simulink model "Wind_Disturbances"  (R2021b)
settings: Solver=VariableStepAuto  StartTime=0.0  StopTime=10.0  RelTol=1e-3
settings Model: Creator=hpShe  LastModifiedBy=hpShe

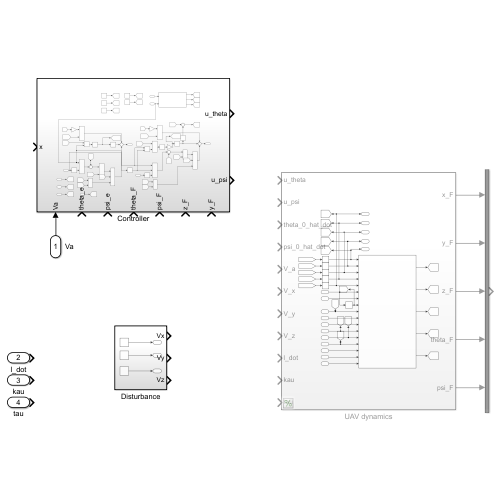
[thumbnail: Simulink's stored preview of the top-level diagram]
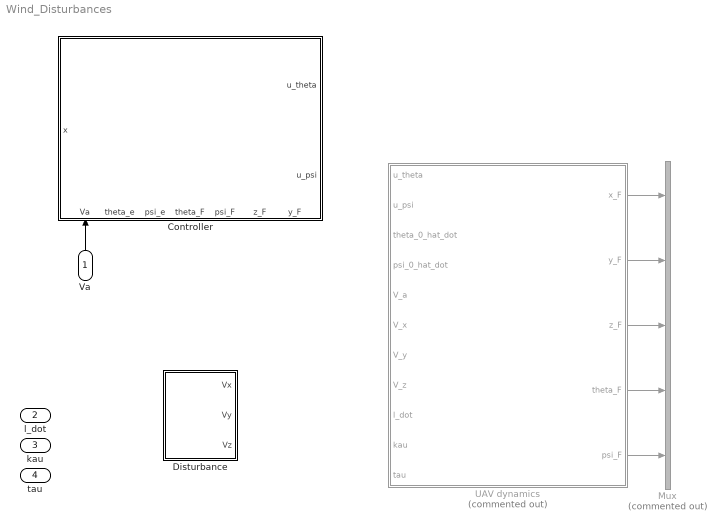
== system Wind_Disturbances ==
  Va : Inport
  l_dot : Inport  Port=2
  kau : Inport  Port=3
  tau : Inport  Port=4
  Controller : Subsystem
      settings: PortSchema="{\"entries\":[{\"content\":{\"sides\":[{\"content\":{\"connectorIds\":[\"In1\"]},\"type\":\"ConnectorPlacement.EquallySpacedRectSide\",\"uuid\":\"85cc706c-7fbb-4ce6-ac6b-8f90726b5cac\"},{\"content\":{\"connectorIds\":[\"Out1\",\"Out2\"],\"side\":\"RIGHT\"},\"type\":\"ConnectorPlacement.EquallySpacedRectSide\",\"uuid\":\"6892ba77-39c0-4603-ac59-cd93350c5557\"},{\"content\":{\"connectorIds\":[],\"side\":\"TOP\"},\"type\":\"ConnectorPlacement.EquallySpacedRectSide\",\"uuid\":\"746b4133-f075-4f92-bb9b-9c21b536ab13\"},{\"content\":{\"connectorIds\":[\"In2\",\"In3\",\"In4\",\"In5\",\"In6\",\"In7\",\"In8\"],\"side\":\"BOTTOM\"},\"type\":\"ConnectorPlacement.EquallySpacedRectSide\",\"uuid\":\"759ff651-9d48-4794-8429-93ccccddab8e\"}]},\"type\":\"ConnectorPlacement.EquallySpacedConnector\",\"uuid\":\"962f8f2c-dfce-46e4-be1a-2f59c37604ab\"}],\"packageUris\":[\"http://schema.mathworks.com/mf0/Connector/R2020b\"],\"version\":\"1.0\"}"
  Disturbance : Subsystem
  Mux : Mux  Commented=on  Inputs=5
  UAV dynamics : Subsystem  Commented=on
  wires:
  Va/1 -> Controller/2(Va)
  UAV dynamics/1(x_F) -> Mux/1
  UAV dynamics/2(y_F) -> Mux/2
  UAV dynamics/3(z_F) -> Mux/3
  UAV dynamics/4(theta_F) -> Mux/4
  UAV dynamics/5(psi_F) -> Mux/5

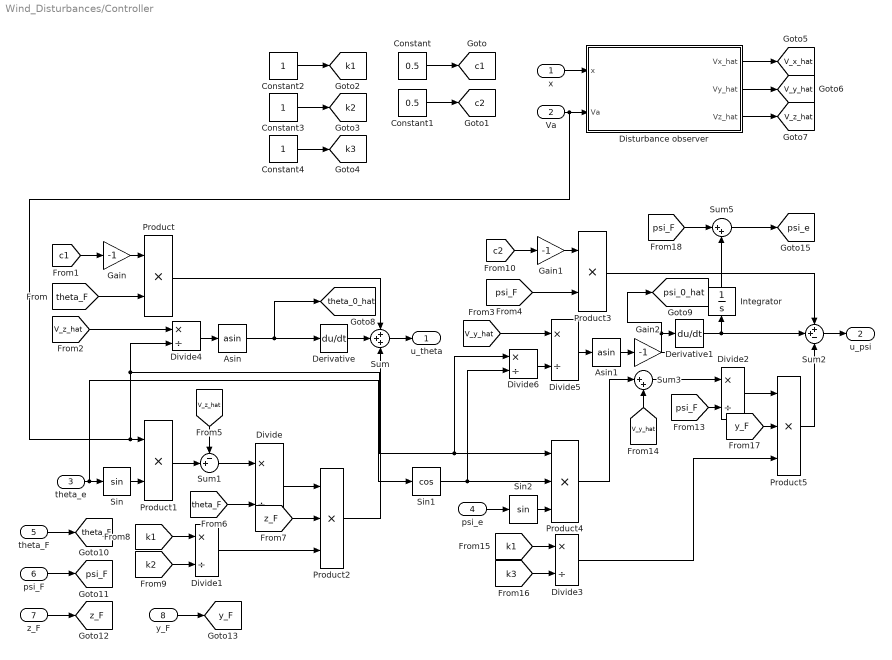
== system Wind_Disturbances/Controller ==
  x : Inport
  Va : Inport  Port=2
  theta_e : Inport  Port=3
  psi_e : Inport  Port=4
  theta_F : Inport  Port=5
  psi_F : Inport  Port=6
  z_F : Inport  Port=7
  y_F : Inport  Port=8
  Asin : Trigonometry  Operator=asin
  Asin1 : Trigonometry  Operator=asin
  Constant : Constant  Value=0.5
  Constant1 : Constant  Value=0.5
  Constant2 : Constant
  Constant3 : Constant
  Constant4 : Constant
  Derivative : Derivative
  Derivative1 : Derivative
  Disturbance observer : Subsystem
  Divide{,1..6} (7 alike) : Product  Inputs=*/
  Gain : Gain  Gain=-1
  Gain1 : Gain  Gain=-1
  Gain2 : Gain  Gain=-1
  Integrator : Integrator
  Product : Product
  Product1 : Product
  Product2 : Product  Inputs=3
  Product3 : Product
  Product4 : Product  Inputs=3
  Product5 : Product  Inputs=3
  Sin : Trigonometry
  Sin1 : Trigonometry  Operator=cos
  Sin2 : Trigonometry
  Sum : Sum  Inputs=+++
  Sum1 : Sum  Inputs=-+|
  Sum2 : Sum  Inputs=++-
  Sum3 : Sum  Inputs=|++
  Sum5 : Sum  Inputs=|++
  u_theta : Outport
  u_psi : Outport  Port=2
  tag scope: V_x_hat=global, V_y_hat=global, V_z_hat=global, c1=global, c2=global, k1=global, k2=global, k3=global, psi_0_hat=global, psi_F=global, psi_e=global, theta_0_hat=global, theta_F=global, y_F=global, z_F=global
  wires:
  [theta_F] -> Product/2
  Constant/1 -> [c1]
  Constant1/1 -> [c2]
  Constant2/1 -> [k1]
  Constant3/1 -> [k2]
  Constant4/1 -> [k3]
  Gain/1 -> Product/1
  [c1] -> Gain/1
  Product/1 -> Sum/1
  Sin/1 -> Product1/2
  Product1/1 -> Sum1/2
  [V_z_hat] -> Sum1/1
  Sum1/1 -> Divide/1
  [theta_F] -> Divide/2
  Divide/1 -> Product2/1
  [z_F] -> Product2/2
  [k1] -> Divide1/1
  [k2] -> Divide1/2
  Divide1/1 -> Product2/3
  Product2/1 -> Sum/3
  Derivative/1 -> Sum/2
  Sum/1 -> u_theta/1
  [psi_F] -> Product3/2
  Product4/1 -> Sum3/1
  Va/1 -> Product4/1, Divide6/1, Divide4/2, Product1/1, Disturbance observer/2(Va)
  [c2] -> Gain1/1
  Sum2/1 -> u_psi/1
  Gain1/1 -> Product3/1
  theta_e/1 -> Sin1/1, Sin/1
  Sin1/1 -> Divide6/2, Product4/2
  Product3/1 -> Sum2/1
  Derivative1/1 -> Integrator/1, Sum2/2
  Sin2/1 -> Product4/3
  [V_y_hat] -> Sum3/2
  Sum3/1 -> Divide2/1
  [psi_F] -> Divide2/2
  Divide2/1 -> Product5/1
  [k3] -> Divide3/2
  [k1] -> Divide3/1
  Divide3/1 -> Product5/3
  [y_F] -> Product5/2
  Product5/1 -> Sum2/3
  [psi_F] -> Sum5/1
  Sum5/1 -> [psi_e]
  Integrator/1 -> Sum5/2
  psi_e/1 -> Sin2/1
  Disturbance observer/1(Vx_hat) -> [V_x_hat]
  Disturbance observer/2(Vy_hat) -> [V_y_hat]
  Disturbance observer/3(Vz_hat) -> [V_z_hat]
  x/1 -> Disturbance observer/1(x)
  Asin/1 -> [theta_0_hat], Derivative/1
  Divide4/1 -> Asin/1
  [V_z_hat] -> Divide4/1
  [V_y_hat] -> Divide5/1
  Divide6/1 -> Divide5/2
  Divide5/1 -> Asin1/1
  Asin1/1 -> Gain2/1
  Gain2/1 -> [psi_0_hat], Derivative1/1
  theta_F/1 -> [theta_F]
  psi_F/1 -> [psi_F]
  z_F/1 -> [z_F]
  y_F/1 -> [y_F]

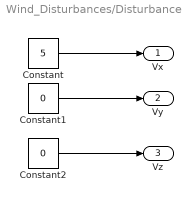
== system Wind_Disturbances/Disturbance ==
  Constant : Constant  Value=5
  Constant1 : Constant  Value=0
  Constant2 : Constant  Value=0
  Vx : Outport
  Vy : Outport  Port=2
  Vz : Outport  Port=3
  wires:
  Constant/1 -> Vx/1
  Constant1/1 -> Vy/1
  Constant2/1 -> Vz/1

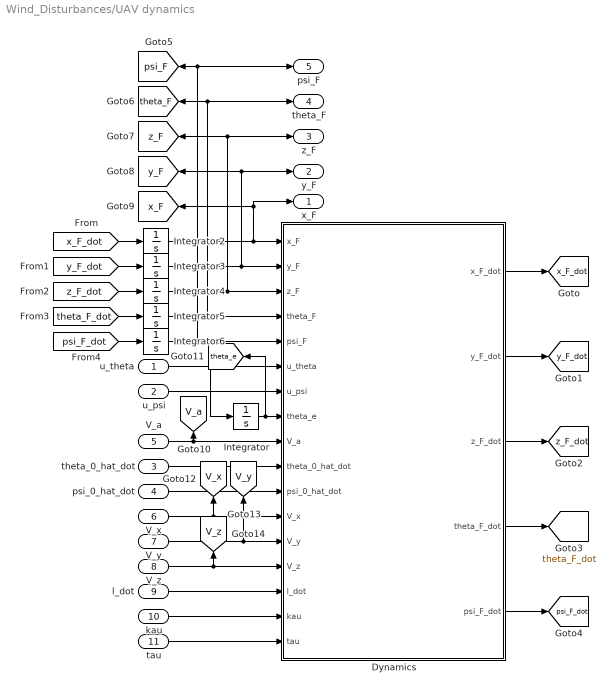
== system Wind_Disturbances/UAV dynamics ==
  u_theta : Inport
  u_psi : Inport  Port=2
  theta_0_hat_dot : Inport  Port=3
  psi_0_hat_dot : Inport  Port=4
  V_a : Inport  Port=5
  V_x : Inport  Port=6
  V_y : Inport  Port=7
  V_z : Inport  Port=8
  l_dot : Inport  Port=9
  kau : Inport  Port=10
  tau : Inport  Port=11
  Dynamics : MATLAB Function  TreatAsAtomicUnit=on
  Integrator{,2..6} (6 alike) : Integrator
  x_F : Outport
  y_F : Outport  Port=2
  z_F : Outport  Port=3
  theta_F : Outport  Port=4
  psi_F : Outport  Port=5
  tag scope: V_a=global, V_x=global, V_y=global, V_z=global, psi_F=global, psi_F_dot=global, theta_F=global, theta_F_dot=global, theta_e=global, x_F=global, x_F_dot=global, y_F=global, y_F_dot=global, z_F=global, z_F_dot=global
  wires:
  l_dot/1 -> Dynamics/15(l_dot)
  [psi_F_dot] -> Integrator6/1
  u_psi/1 -> Dynamics/7(u_psi)
  kau/1 -> Dynamics/16(kau)
  V_z/1 -> [V_z], Dynamics/14(V_z)
  [y_F_dot] -> Integrator3/1
  psi_0_hat_dot/1 -> Dynamics/11(psi_0_hat_dot)
  tau/1 -> Dynamics/17(tau)
  [z_F_dot] -> Integrator4/1
  Dynamics/4(theta_F_dot) -> [theta_F_dot]
  [x_F_dot] -> Integrator2/1
  V_x/1 -> [V_x], Dynamics/12(V_x)
  Integrator3/1 -> [y_F], y_F/1, Dynamics/2(y_F)
  u_theta/1 -> Integrator/1, Dynamics/6(u_theta)
  V_y/1 -> [V_y], Dynamics/13(V_y)
  Integrator4/1 -> [z_F], z_F/1, Dynamics/3(z_F)
  Integrator5/1 -> theta_F/1, [theta_F], Dynamics/4(theta_F)
  Dynamics/5(psi_F_dot) -> [psi_F_dot]
  Integrator2/1 -> [x_F], x_F/1, Dynamics/1(x_F)
  Integrator/1 -> [theta_e], Dynamics/8(theta_e)
  Dynamics/3(z_F_dot) -> [z_F_dot]
  Dynamics/2(y_F_dot) -> [y_F_dot]
  Dynamics/1(x_F_dot) -> [x_F_dot]
  theta_0_hat_dot/1 -> Dynamics/10(theta_0_hat_dot)
  [theta_F_dot] -> Integrator5/1
  V_a/1 -> [V_a], Dynamics/9(V_a)
  Integrator6/1 -> [psi_F], psi_F/1, Dynamics/5(psi_F)

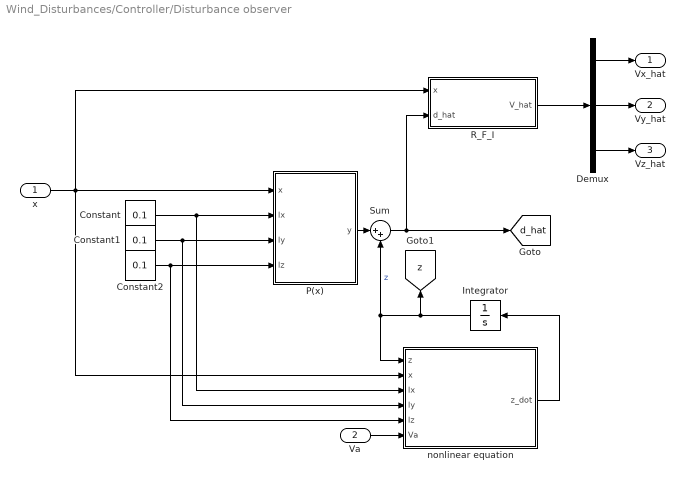
== system Wind_Disturbances/Controller/Disturbance observer ==
  x : Inport
  Va : Inport  Port=2
  Constant : Constant  Value=0.1
  Constant1 : Constant  Value=0.1
  Constant2 : Constant  Value=0.1
  Demux : Demux  Outputs=3
  Integrator : Integrator
  P(x) : MATLAB Function  TreatAsAtomicUnit=on
  R_F_I : MATLAB Function  TreatAsAtomicUnit=on
  Sum : Sum  Inputs=|++
  nonlinear equation : MATLAB Function  TreatAsAtomicUnit=on
  Vx_hat : Outport
  Vy_hat : Outport  Port=2
  Vz_hat : Outport  Port=3
  tag scope: d_hat=global, z=global
  wires:
  x/1 -> P(x)/1(x), nonlinear equation/2(x), R_F_I/1(x)
  P(x)/1(y) -> Sum/1
  Sum/1 -> R_F_I/2(d_hat), [d_hat]
  nonlinear equation/1(z_dot) -> Integrator/1
  Integrator/1 -> [z], nonlinear equation/1(z), Sum/2  "z"
  R_F_I/1(V_hat) -> Demux/1
  Demux/1 -> Vx_hat/1
  Demux/2 -> Vy_hat/1
  Demux/3 -> Vz_hat/1
  Constant/1 -> nonlinear equation/3(lx), P(x)/2(lx)
  Constant1/1 -> nonlinear equation/4(ly), P(x)/3(ly)
  Constant2/1 -> nonlinear equation/5(lz), P(x)/4(lz)
  Va/1 -> nonlinear equation/6(Va)

== matlab function Wind_Disturbances/UAV dynamics/Dynamics ==
  data: x_F input; x_F_dot output; y_F_dot output; z_F_dot output; theta_F_dot output; psi_F_dot output; y_F input; z_F input; theta_F input; psi_F input; u_theta input; u_psi input; theta_e input; V_a input; theta_0_hat_dot input; psi_0_hat_dot input; V_x input; V_y input; V_z input; l_dot input; kau input; tau input
function [x_F_dot,y_F_dot,z_F_dot,theta_F_dot,psi_F_dot] = fcn( x_F,y_F,z_F,theta_F,psi_F,...
                                                                u_theta,u_psi, theta_e, ...
                                                                V_a, ...
                                                                theta_0_hat_dot, psi_0_hat_dot, ...
                                                                V_x,V_y,V_z, ...
                                                                l_dot,kau,tau)
    theta_0 = asin(V_z/V_a);
    
    psi_0 = -asin(V_y/(V_a * cos(theta_e))); 

    x_F_dot = V_a * cos(theta_F + theta_0) * cos(psi_F + psi_0) - l_dot * (1-kau * y_F) + V_x;

    y_F_dot = V_a * cos(theta_F + theta_0) * sin(psi_F + psi_0) - l_dot * (kau *x_F - tau * z_F) + V_y;

    z_F_dot = -V_a * sin(theta_F + theta_0) - l_dot * tau * y_F + V_z;

    theta_F_dot = u_theta - theta_0_hat_dot;

    psi_F_dot = u_psi - psi_0_hat_dot;

end

== matlab function Wind_Disturbances/Controller/Disturbance observer/P(x) ==
  data: x input; y output; lx input; ly input; lz input
function y = P(x,lx,ly,lz)

    X = x(1);
    Y = x(2);
    Z = x(3);
    theta = x(4);
    psi = x(5);

    y = [lx * X; ly * Y; lz * Z];

end

== matlab function Wind_Disturbances/Controller/Disturbance observer/nonlinear equation ==
  data: z input; x input; z_dot output; lx input; ly input; lz input; Va input
function z_dot = nonlinear_equation(z,x,lx,ly,lz,Va)

    X = x(1);
    Y = x(2);
    Z = x(3);
    theta = x(4);
    psi = x(5);

    p_x = [lx * X; ly * Y; lz * Z];
    
    g_2_x = diag([1 1 1]);

    l_x = diag([lx ly lz]);

    f_x = [ Va * cos(theta) * cos(psi);...
            Va * cos(theta) * sin(psi);...
           -Va * sin(theta)];


    z_dot = - l_x * g_2_x * z - l_x * (f_x + g_2_x * p_x);

end

== matlab function Wind_Disturbances/Controller/Disturbance observer/R_F_I ==
  data: x input; V_hat output; d_hat input
function V_hat = R_F_I(x,d_hat)

    y = u;

end
